simulink model "crazy_model_linearize"  (R2014b)
settings: Solver=ode4  StartTime=0.0  StopTime=10  FixedStep=0.01  RelTol=1e-3
values from neighbouring files (symbols this model uses):
  Kv = 14000*[1 0 0 0 ... (first row only)    [control_PWM.m]    (also in linearize_pwm.m = 14000; linearize_voltage.m = 14000; main.m = 14000)
settings Model: Creator=Abhiram  LastModifiedBy=Abhiram

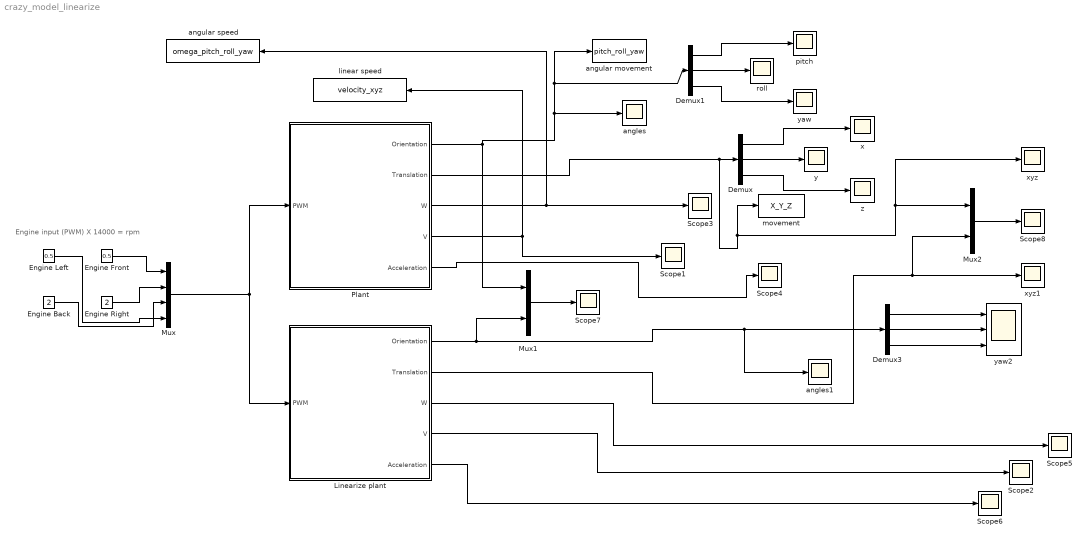
== system crazy_model_linearize ==
  note: Engine input (PWM) X 14000 = rpm
  Demux : Demux  Outputs=3
  Demux1 : Demux  Outputs=3
  Demux3 : Demux  Outputs=3
  Engine Back : Constant  Value=2
  Engine Front : Constant  Value=0.5
  Engine Left : Constant  Value=0.5
  Engine Right : Constant  Value=2
  Linearize plant : Subsystem
  Mux : Mux
  Mux1 : Mux  Inputs=2
  Mux2 : Mux  Inputs=2
  Plant : Subsystem
  Scope{1..8} (8 alike) : Scope
      Scope2 settings: SaveName=ScopeData11
      Scope3 settings: SaveName=ScopeData3
      Scope4 settings: SaveName=ScopeData4
      Scope5 settings: SaveName=ScopeData12
      Scope6 settings: SaveName=ScopeData13
      Scope7 settings: SaveName=ScopeData18
      Scope8 settings: SaveName=ScopeData20
  angles : Scope
      settings: SaveName=ScopeData10
  angles1 : Scope
      settings: SaveName=ScopeData14
  angular movement : ToWorkspace  VariableName=pitch_roll_yaw  SaveFormat=Structure With Time  SampleTime=-1
  angular speed : ToWorkspace  VariableName=omega_pitch_roll_yaw  SaveFormat=Structure With Time  SampleTime=-1
  linear speed : ToWorkspace  VariableName=velocity_xyz  SaveFormat=Structure With Time  SampleTime=-1
  movement : ToWorkspace  VariableName=X_Y_Z  SaveFormat=Structure With Time  SampleTime=-1
  pitch : Scope
  roll : Scope
      settings: TimeRange=10  YMin=0  YMax=25  SaveName=ScopeData7
  x : Scope
      settings: SaveName=ScopeData2
  xyz : Scope
      settings: TimeRange=10  YMin=-20  YMax=120  SaveName=ScopeData9
  xyz1 : Scope
      settings: TimeRange=10  YMin=-20  YMax=120  SaveName=ScopeData17
  y : Scope
      settings: SaveName=ScopeData5
  yaw : Scope
      settings: SaveName=ScopeData8
  yaw2 : Scope  NumInputPorts=3
      settings: YMin=-5~-5~-5  YMax=5~5~5  SaveName=ScopeData21
  z : Scope
      settings: SaveName=ScopeData6
  wires:
  Plant/1(Orientation) -> angular movement/1, Demux1/1, angles/1, Mux1/1
  Plant/3(W) -> angular speed/1, Scope3/1
  Plant/4(V) -> linear speed/1, Scope1/1
  Plant/5(Acceleration) -> Scope4/1
  Plant/2(Translation) -> Demux/1, movement/1, xyz/1, Mux2/1
  Demux/1 -> x/1
  Demux/2 -> y/1
  Demux/3 -> z/1
  Demux1/1 -> pitch/1
  Demux1/2 -> roll/1
  Demux1/3 -> yaw/1
  Mux/1 -> Plant/1(PWM), Linearize plant/1(PWM)
  Linearize plant/1(Orientation) -> Mux1/2, angles1/1, Demux3/1
  Linearize plant/3(W) -> Scope5/1
  Linearize plant/4(V) -> Scope2/1
  Linearize plant/5(Acceleration) -> Scope6/1
  Linearize plant/2(Translation) -> xyz1/1, Mux2/2
  Demux3/1 -> yaw2/1
  Demux3/2 -> yaw2/2
  Mux1/1 -> Scope7/1
  Mux2/1 -> Scope8/1
  Demux3/3 -> yaw2/3
  Engine Front/1 -> Mux/1
  Engine Right/1 -> Mux/2
  Engine Back/1 -> Mux/3
  Engine Left/1 -> Mux/4

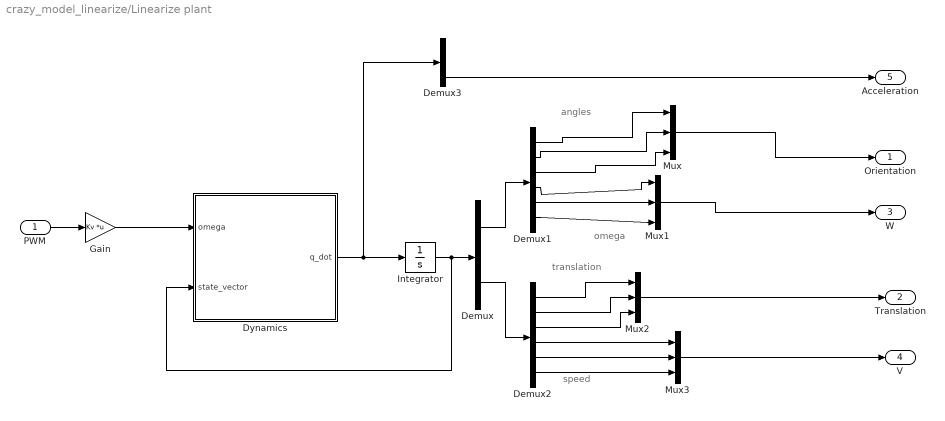
== system crazy_model_linearize/Linearize plant ==
  note: speed
  note: translation
  note: omega
  note: angles
  PWM : Inport
  Demux : Demux  Outputs=2
  Demux1 : Demux  Outputs=6
  Demux2 : Demux  Outputs=6
  Demux3 : Demux
  Dynamics : MATLAB Function  TreatAsAtomicUnit=on
  Gain : Gain  Gain=Kv  Multiplication=Matrix(K*u)
  Integrator : Integrator  InitialCondition=[0 0 0 0 0 0 0 0 0 0 0 0]'
  Mux{,1..3} (4 alike) : Mux  Inputs=3
  Orientation : Outport
  Translation : Outport  Port=2
  W : Outport  Port=3
  V : Outport  Port=4
  Acceleration : Outport  Port=5
  wires:
  PWM/1 -> Gain/1
  Gain/1 -> Dynamics/1(omega)
  Dynamics/1(q_dot) -> Demux3/1, Integrator/1
  Integrator/1 -> Dynamics/2(state_vector), Demux/1
  Demux/1 -> Demux1/1
  Demux/2 -> Demux2/1
  Demux1/5 -> Mux1/2
  Demux1/6 -> Mux1/3
  Demux1/4 -> Mux1/1
  Demux1/1 -> Mux/1
  Demux1/2 -> Mux/2
  Demux1/3 -> Mux/3
  Demux2/5 -> Mux3/2
  Demux2/6 -> Mux3/3
  Demux2/4 -> Mux3/1
  Demux2/1 -> Mux2/1
  Demux2/2 -> Mux2/2
  Demux2/3 -> Mux2/3
  Mux/1 -> Orientation/1
  Mux1/1 -> W/1
  Mux2/1 -> Translation/1
  Mux3/1 -> V/1
  Demux3/4 -> Acceleration/1

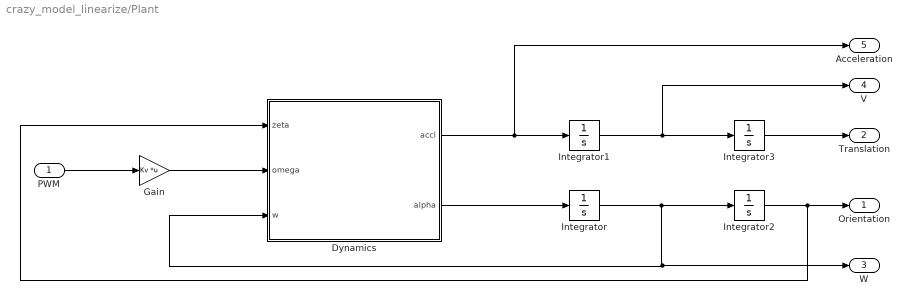
== system crazy_model_linearize/Plant ==
  PWM : Inport
  Dynamics : MATLAB Function  TreatAsAtomicUnit=on
  Gain : Gain  Gain=Kv  Multiplication=Matrix(K*u)
  Integrator{,1..3} (4 alike) : Integrator  InitialCondition=[0 0 0]'
  Orientation : Outport
  Translation : Outport  Port=2
  W : Outport  Port=3
  V : Outport  Port=4
  Acceleration : Outport  Port=5
  wires:
  Integrator/1 -> Integrator2/1, Dynamics/3(w), W/1
  Integrator1/1 -> V/1, Integrator3/1
  Integrator2/1 -> Dynamics/1(zeta), Orientation/1
  Integrator3/1 -> Translation/1
  PWM/1 -> Gain/1
  Dynamics/2(alpha) -> Integrator/1
  Dynamics/1(accl) -> Acceleration/1, Integrator1/1
  Gain/1 -> Dynamics/2(omega)

== matlab function crazy_model_linearize/Linearize plant/Dynamics ==
  data: omega input; state_vector input; q_dot output
function q_dot  = fcn(omega, state_vector)

    Ixx = 2.09*10^(-05);
    Iyy = 2.09*10^(-05);
    Izz = 3.81*10^(-05);
    I = diag([Ixx,Iyy,Izz]);                                            % Inertia matrix - needs revision

    d = 0.046;
    m = 0.027;
    g = 9.8;
    
    zeta = state_vector(1:3);
    w = state_vector(4:6);
    trans = state_vector(7:9);
    speeds = state_vector(10:12);
    
    theta = zeta(1);                                                    % pitch    
    phi = zeta(2);                                                      % roll
    psi = zeta(3);                                                      % yaw
    
    u = thrust(omega);
    operating_q = state_vector;
    operating_u = thrust(omega);
    
    [A,B,constant] = linearize(operating_q, operating_u);
    
    q_dot = A*state_vector + B*u + constant;
       
end

== matlab function crazy_model_linearize/Plant/Dynamics ==
  data: zeta input; omega input; accl output; alpha output; w input
function [accl, alpha] = fcn(zeta, omega, w)

    Ixx = 2.09*10^(-05);
    Iyy = 2.09*10^(-05);
    Izz = 3.81*10^(-05);
    I = diag([Ixx,Iyy,Izz]);                              % Inertia matrix - needs revision

%   Ct = 10;
%   Cq = 10;
    d = 0.046;
    m = 0.027;
    g = 9.8;
    % Inertia = ?

%%%%%%%%%%%%%%%%%%%%%%%%%%%%%%%%%%%%%%%%%%%%%%%%%%%%%%%%%%%%%%%%%%%%%%%%%%%
%3
    theta = zeta(1);         % pitch    
    phi = zeta(2);           % roll
    psi = zeta(3);           % yaw
    
    [T_b] = thrust(omega);              % non linear function for thrust
    
    F_e = T_b(1)*[-sin(theta); cos(theta)*sin(phi); cos(theta)*cos(phi)];
    
    Tau_e = [T_b(2) T_b(3) T_b(4)]';
    G = [0 0 m*g]';

    T_e = [F_e - G; Tau_e];

    I_a = [m*eye(3)    zeros(3,3);
           zeros(3,3)         I ];

    w_cross = cross(w,I*w);

    % Needs Revision
    A = I_a \ ( T_e - [0;0;0;w_cross] );
    
    accl = A(1:3);
    alpha = A(4:6);

end
